simulink library "neural"  (Simulink 5.0)
undefined symbols (not defined in the file or in its folder): sfunxy2
libraries: simulink3 x7
settings Model: Creator=mani  LastModifiedBy=munlock -all d:\work\myr12\toolbox\fuzzy\fuzzy\mfedit.m

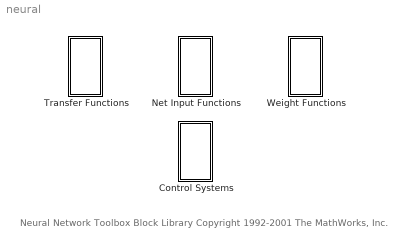
== system neural ==
  note: Neural Network Toolbox Block Library
      | Copyright 1992-2001 The MathWorks, Inc.
  Control Systems : Subsystem
      settings: RTWFcnNameOpts=Auto  RTWFileNameOpts=Auto
  Net Input Functions : Subsystem
      settings: RTWFcnNameOpts=Auto  RTWFileNameOpts=Auto
  Transfer Functions : Subsystem
      settings: RTWFcnNameOpts=Auto  RTWFileNameOpts=Auto
  Weight Functions : Subsystem
      settings: RTWFcnNameOpts=Auto  RTWFileNameOpts=Auto

== system neural/Control Systems ==
  Model Reference Controller : Subsystem  mask(NN Model Reference Control){Nrc=, Nic=, Njc=, IW_y=, IW_u=, IW_r=, B1_c=, B2_c=, LW_c=, retraining_c=, max_i_int=, min_i_int=, max_r_int=, min_r_int=, Ts=, S1=, Ni=, Nj=, sim_file=, trainfun=trainlm, Use_validation=, Use_Testing=, Use_Inc_training=, Use_previous_weights=, max_i=, min_i=, max_r=, min_r=, sam_training=, sam_training_c=, epochs=, epochs_c=, minp=, maxp=, mint=, maxt=, Normalize=, IW=, LW1_2=, LW2_1=, B1=, B2=, S1c=, Limit_output=, min_output=, max_output=, Ref_file=}
      mask prompts: Ts "Sample time"; trainfun "Training function Identification"; Limit_output "Limit output"
      mask help: Neural network model reference controller. You first train a neural network model of the plant to be controlled. Then train the controller so that the plant output will follow the output of a reference model. Double-click the Model Reference Control block to begin the plant and controller training.
      mask init:
      | xl = [0   .53     .53     .92   .92   .53   .53  NaN ];
      | yl = [.95 .95 1.05 1.05 .3   .3   .95 NaN  ];
      | x2 = [0 .53    NaN .92 1.2  ];
      | y2 = [.39 .39   NaN .65 .65  ];
      | t=(0:24)/24*2*pi;
      | xs = .07*cos(t)+.9;
      | ys = .07*sin(t)+.75;
      | 
      | x1t=.03; y1t=.31;
      | x2t=.03; y2t=.8;
      | x3t=.77; y3t=.53;
      | x4t=.77; y4t=.44;
      | x5t=.45; y5t=.66;
      | x6t=.45; y6t=.55;
      | x7t=.45; y7t=.44;
      settings: OpenFcn=nncontrolutil('nnmodref','',gcbh,gcb,'');  RTWFcnNameOpts=Auto  RTWFileNameOpts=Auto
      mask Help: eval('nnetbhelp([],''contro10.html'')');
      mask StyleString: edit,edit,edit,edit,edit,edit,edit,edit,edit,edit,edit,edit,edit,edit,edit,edit,edit,edit,edit,popup(trainbfg|trainbr |traincgb|traincgf|traincgp|traingd|traingdm|traingda|traingdx|trainlm |trainoss|trainrp |trainscg),edit,edit,edit,edit,edit,edit,edit,edit,edit,edit,edit,edit,edit,edit,edit,edit,edit,edit,edit,edit,edit,edit,edit,edit,edit,edit,edit
      mask Display:
      | plot([[xl NaN x2]*.9-.075 ], [[yl  NaN y2]*.9-.1 ]);
      | text(x1t,y1t,'Plant Output');
      | text(x2t,y2t,'Reference');
      | text(x3t,y3t,'Control');
      | text(x4t,y4t,'Signal');
      | text(x5t,y5t,'Neural');
      | text(x6t,y6t,'Network');
      | text(x7t,y7t,'Controller');
  NARMA-L2 Controller : Subsystem  mask(NARMA-L2 Controller){Normalize=, IW1_1=, IW3_2=, IW5_3=, LW2_1=, LW4_3=, LW5_4=, LW6_5=, LW6_2=, B1=, B2=, B3=, B4=, Limit_output=, min_output=, max_output=, Use_Previous_Weights=, Ts=, S1=, Ni=, Nj=, sim_file=, trainfun=trainlm, Use_validation=, Use_Testing=, max_i=, min_i=, max_i_int=, min_i_int=, sam_training=, epochs=, minp=, maxp=, mint=, maxt=}
      mask prompts: Ts "Sample time"; trainfun "Training function"
      mask help: NARMA-L2 Controller. You first train a neural network model of the plant to be controlled. The controller is a rearrangement of the trained plant model. Double-click the NARMA-L2 Controller block to begin the plant training.
      mask init:
      | xl = [0    .4   NaN  .33  .55   .55  .33  .33  NaN .80  .92 .92];
      | yl = [.95 .95 NaN  .75  .75   .55  .55  .75  NaN  .95 .95 .65];
      | x2 = [0    .43 NaN .45 .45    NaN .92 1.2 NaN .63 .85 .85 .63 .63 ];
      | y2 = [.39 .39 NaN  .41 .55   NaN .65 .65 NaN .75 .75  .55  .55  .75];
      | x3 = [.45 .45 NaN .42 .45 .48  NaN .33 .4 .33];
      | y3 = [.75 .90 NaN .83 .90 .83  NaN  .98 .95 .92];
      | x4 = [.75 .75 NaN .72 .75 .78  NaN  .5 .7 NaN .63 .7 .63];
      | y4 = [.75 .90 NaN .83 .90 .83  NaN .95 .95 NaN .98 .95 .92];
      | x5 = [.43 .43 .77 .77 .43 NaN .36 .43 .36 NaN .75 .75];
      | y5 = [.37 .41 .41 .37 .37 NaN .42 .39 .36 NaN .41 .55];
      | x6 = [.92 .92 .77 NaN .84 .77 .84];
      | y6 = [.65 .39 .39 NaN .42 .39 .36];
      | x1t=.03; y1t=.31;
      | x2t=.03; y2t=.85;
      | x8t=.03;y8t=.21;
      | x3t=.77; y3t=.53;
      | x4t=.77; y4t=.44;
      | x5t=.34; y5t=.49;
      | x6t=.58; y6t=.49;
      | 
      | 
      | t=(0:24)/24*2*pi;
      | xs = .05*cos(t);
      | ys = .05*sin(t);
      | xs1=xs+.45;
      | ys1=ys+.95;
      | xs2=xs+.75;
      | ys2=ys+.95;
      settings: OpenFcn=nncontrolutil('nnident','',gcbh,gcb,'narma_l2');  RTWFcnNameOpts=Auto  RTWFileNameOpts=Auto
      mask Help: eval('nnetbhelp([],''contro6a.html'')');
      mask StyleString: edit,edit,edit,edit,edit,edit,edit,edit,edit,edit,edit,edit,edit,edit,edit,edit,edit,edit,edit,edit,edit,edit,popup(trainbfg|trainbr |traincgb|traincgf|traincgp|traingd|traingdm|traingda|traingdx|trainlm |trainoss|trainrp |trainscg),edit,edit,edit,edit,edit,edit,edit,edit,edit,edit,edit,edit
      mask Display:
      | plot([[xl NaN x2]*.9-.075 ], [[yl  NaN y2]*.9-.1 ]);
      | plot([[x3 NaN xs1 NaN xs2]*.9-.075 ], [[y3 NaN ys1 NaN ys2]*.9-.1 ]);
      | plot([x4 NaN x5]*.9-.075,[y4 NaN y5]*.9-.1);
      | plot([x6 NaN ]*.9-.075,[y6 NaN ]*.9-.1);
      | text(x1t,y1t,'Plant');
      | text(x8t,y8t,'Output');
      | text(x2t,y2t,'Reference');
      | text(x3t,y3t,'Control');
      | text(x4t,y4t,'Signal');
      | text(x5t,y5t,'f');
      | text(x6t,y6t,'g');
  NN Predictive Controller : Subsystem  mask(NN Predictive Controller){epochs=, minp=, maxp=, mint=, maxt=, Normalize=, IW=, LW1_2=, LW2_1=, B1=, B2=, max_i_int=, min_i_int=, limit_output=, max_output=, min_output=, Use_Previous_Weights=, N2=, Nu=, Ts=, rho=, alpha=, csrchfun=csrchbac, maxiter=, S1=, Ni=, Nj=, sim_file=, trainfun=trainlm, Use_validation=, Use_Testing=, max_i=, min_i=, sam_training=}
      mask prompts: Ts "Sample time"; rho "rho (typically = 0.03)"; alpha "alpha (typically = 0.001)"; csrchfun "Minimization rutine"; trainfun "Training function"
      mask help: NN Predictive Controller. You first train a neural network model of the plant to be controlled. The controller uses the plant model to predict plant performance over a specified time horizon. An optimization algorithm determines the control signal that optimizes plant performance over this horizon. Double click the NN Predictive Controller block to train the plant model and set the controller parameters.
      mask init:
      | xl = [0   .53   .53     .85   .85  .53  .53  NaN .85  .92 .92];
      | yl = [.95 .95 1.05  1.05   .82  .82  .95  NaN  .95 .95 .65];
      | x2 = [0 .53    NaN .92 1.2 NaN .53 .85 .85 .53 .53 ];
      | y2 = [.39 .39   NaN .65 .65 NaN .59 .59 .29 .29  .59];
      | x3 = [.67 .67 NaN .64 .67 .70 NaN .53 .4   .4   .53 NaN .46 .53 .46];
      | y3 = [.59 .82 NaN .66 .59 .66 NaN .55 .55 .86 .86 NaN  .89 .86 .83];
      | 
      | x1t=.03; y1t=.31;
      | x2t=.03; y2t=.8;
      | x8t=.03;y8t=.21;
      | x3t=.77; y3t=.53;
      | x4t=.77; y4t=.44;
      | x5t=.45; y5t=.76;
      | x6t=.45; y6t=.35;
      | x7t=.45; y7t=.25;
      settings: OpenFcn=nncontrolutil('nnpredict','',gcbh,gcb);  RTWFcnNameOpts=Auto  RTWFileNameOpts=Auto
      mask Help: eval('nnetbhelp([],''control2.html'')');
      mask StyleString: edit,edit,edit,edit,edit,edit,edit,edit,edit,edit,edit,edit,edit,edit,edit,edit,edit,edit,edit,edit,edit,edit,popup(csrchgol|csrchbac|csrchhyb|csrchbre|csrchcha),edit,edit,edit,edit,edit,popup(trainbfg|trainbr |traincgb|traincgf|traincgp|traingd|traingdm|traingda|traingdx|trainlm |trainoss|trainrp |trainscg),edit,edit,edit,edit,edit
      mask Display:
      | plot([[xl NaN x2]*.9-.075 ], [[yl  NaN y2]*.9-.1 ]);
      | plot([[x3]*.9-.075 ], [[y3]*.9-.1 ]);
      | text(x1t,y1t,'Plant');
      | text(x8t,y8t,'Output');
      | text(x2t,y2t,'Reference');
      | text(x3t,y3t,'Control');
      | text(x4t,y4t,'Signal');
      | text(x5t,y5t,'Optim.');
      | text(x6t,y6t,'NN');
      | text(x7t,y7t,'Model');
  X(2Y)  Graph : Subsystem  LoadFcn=sfunxy2([],[],[],'LoadBlock')  StartFcn=sfunxy2([],[],[],'Start')  StopFcn=sfunxy2([],[],[],'Stop')  mask(X(2Y) scope.){xmin=0, xmax=5, ymin=21, ymax=22, st=-1}
      mask prompts: xmin "x-min:"; xmax "x-max:"; ymin "y-min:"; ymax "y-max:"; st "Sample time:"
      mask help: X(2Y) scope using MATLAB graph window. First input is used as time base. Enter plotting ranges.
      settings: CopyFcn=sfunxy2([],[],[],'CopyBlock')  DeleteFcn=sfunxy2([],[],[],'DeleteBlock')  NameChangeFcn=sfunxy2([],[],[],'NameChange')  RTWFcnNameOpts=Auto  RTWFileNameOpts=Auto
      mask Help: This block can be used to explore limit cycles. Look at the m-file sfunxy.m to see how it works.
      mask Display: plot([.05 .95 .95 .05 .05],[.45 .45 .95 .95 .45], 0.5+cos(0:0.1:2*pi)*0.3,0.7+sin(0:0.1:2*pi)*0.2)

== system neural/Net Input Functions ==
  netprod : Product  Inputs=2  Multiplication=Element-wise(.*)  SaturateOnIntegerOverflow=on
  netsum : Sum  Inputs=2  SaturateOnIntegerOverflow=on

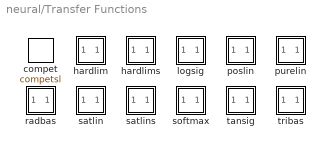
== system neural/Transfer Functions ==
  compet : MATLABFcn  MATLABFcn=competsl  OutputDimensions=-1  OutputSignalType=auto  Output1D=on
      mask Type: compet
      mask Description: Competitive transfer function
      mask Help: eval('nnetbhelp(''compet'')');
      mask Display: disp('C')
  hardlim : Subsystem
      settings: RTWFcnNameOpts=Auto  RTWFileNameOpts=Auto
      mask Type: Hardlim
      mask Description: Hard limit transfer function
      mask Help: eval('nnetbhelp(''hardlim'')');
      mask Display: plot([-1 1],[-1 -1],[-1 0 0 1],[-1 -1 1 1])
  hardlims : Subsystem
      settings: RTWFcnNameOpts=Auto  RTWFileNameOpts=Auto
      mask Description: Symmetric hard limit transfer function
      mask Help: eval('nnetbhelp(''hardlims'')');
      mask Display: plot([-1 1],[0 0],[-1 0 0 1],[-1 -1 1 1])
  logsig : Subsystem
      settings: RTWFcnNameOpts=Auto  RTWFileNameOpts=Auto
      mask Description: Log sigmoid transfer function
      mask Help: eval('nnetbhelp(''logsig'')');
      mask Display: plot([-1 1],[0 0],[-1 -.9 -.8 -.7 -.6 -.5 -.4 -.3 -.2 -.1 0 .1 .2 .3 .4 .5 .6 .7 .8 .9 1],1./(1+exp(-8*[-1 -.9 -.8 -.7 -.6 -.5 -.4 -.3 -.2 -.1 0 .1 .2 .3 .4 .5 .6 .7 .8 .9 1]))+.01)
  poslin : Subsystem  Orientation=left
      settings: RTWFcnNameOpts=Auto  RTWFileNameOpts=Auto
      mask Description: Positive linear transfer function
      mask Help: eval('nnetbhelp(''poslin'')');
      mask Display: plot([-1 1],[-1 -1],[-1 -.5 1],[-1 -1 1])
  purelin : Subsystem
      settings: RTWFcnNameOpts=Auto  RTWFileNameOpts=Auto
      mask Description: Linear transfer function
      mask Help: eval('nnetbhelp(''purelin'')');
      mask Display: plot([-1 1],[0 0],[-1 1],[-1 1])
  radbas : Subsystem
      settings: RTWFcnNameOpts=Auto  RTWFileNameOpts=Auto
      mask Description: Radial basis transfer function
      mask Help: eval('nnetbhelp(''radbas'')');
      mask Display: plot([-1 1],[0 0],[-1 -.9 -.8 -.7 -.6 -.5 -.4 -.3 -.2 -.1 0 .1 .2 .3 .4 .5 .6 .7 .8 .9 1],exp(-4*([-1 -.9 -.8 -.7 -.6 -.5 -.4 -.3 -.2 -.1 0 .1 .2 .3 .4 .5 .6 .7 .8 .9 1].^2)))
  satlin : Subsystem
      settings: RTWFcnNameOpts=Auto  RTWFileNameOpts=Auto
      mask Description: Saturating linear transfer function
      mask Help: eval('nnetbhelp(''satlin'')');
      mask Display: plot([-1 1],[-1 -1],[-1 -0.5 0.5 1],[-1 -1 1 1])
  satlins : Subsystem
      settings: RTWFcnNameOpts=Auto  RTWFileNameOpts=Auto
      mask Description: Symmetric saturating linear transfer function
      mask Help: eval('nnetbhelp(''satlins'')');
      mask Display: plot([-1 1],[0 0],[-1 -0.5 0.5 1],[-1 -1 1 1])
  softmax : Subsystem
      settings: RTWFcnNameOpts=Auto  RTWFileNameOpts=Auto
      mask Description: Soft max transfer function
      mask Help: eval('nnetbhelp(''softmax'')');
      mask Display: disp('S')
  tansig : Subsystem
      settings: RTWFcnNameOpts=Auto  RTWFileNameOpts=Auto
      mask Description: Hyperbolic tangent sigmoid transfer function
      mask Help: eval('nnetbhelp(''tansig'')');
      mask Display: plot([-1 1],[0 0],[-1 -.9 -.8 -.7 -.6 -.5 -.4 -.3 -.2 -.1 0 .1 .2 .3 .4 .5 .6 .7 .8 .9 1],2./(1+exp(-8*[-1 -.9 -.8 -.7 -.6 -.5 -.4 -.3 -.2 -.1 0 .1 .2 .3 .4 .5 .6 .7 .8 .9 1]))-1)
  tribas : Subsystem
      settings: RTWFcnNameOpts=Auto  RTWFileNameOpts=Auto
      mask Description: Triangular basis transfer function
      mask Help: eval('nnetbhelp(''tribas'')');
      mask Display: plot([-1 1],[0 0],[-1 -.6 0 .6 1],[0 0 1 0 0])

== system neural/Weight Functions ==
  dist : Subsystem
      settings: RTWFcnNameOpts=Auto  RTWFileNameOpts=Auto
      mask Description: Euclidean distance weight function
      mask Help: eval('nnetbhelp(''dist'')');
  dotprod : Subsystem
      settings: RTWFcnNameOpts=Auto  RTWFileNameOpts=Auto
      mask Description: Dot product weight function
      mask Help: eval('nnetbhelp(''dotprod'')');
  negdist : Subsystem
      settings: RTWFcnNameOpts=Auto  RTWFileNameOpts=Auto
      mask Description: The negative of the euclidean distance weight function
      mask Help: eval('nnetbhelp(''negdist'')');
  normprod : Subsystem
      settings: RTWFcnNameOpts=Auto  RTWFileNameOpts=Auto
      mask Description: Normalized dot product weight function
      mask Help: eval('nnetbhelp(''normprod'')');

== system neural/Control Systems/Model Reference Controller ==
  Reference : Inport  Port=1  LatchInput=off
  Plant Output : Inport  Orientation=up  Port=2  LatchInput=off
  NN Controller : Subsystem
      settings: RTWFcnNameOpts=Auto  RTWFileNameOpts=Auto
  NN Plant : Subsystem
      settings: RTWFcnNameOpts=Auto  RTWFileNameOpts=Auto
  Terminator : Terminator
  Terminator1 : Terminator
  Control Signal : Outport  Orientation=down  Port=1
  wires:
  NN Plant/2(yhat1) -> Terminator1/1
  NN Plant/1(yhat) -> Terminator/1
  Reference/1 -> NN Controller/1(r)
  NN Controller/1(uhat) -> NN Controller/2(u), Control Signal/1, NN Plant/1(u)
  Plant Output/1 -> NN Controller/3(y), NN Plant/2(y)

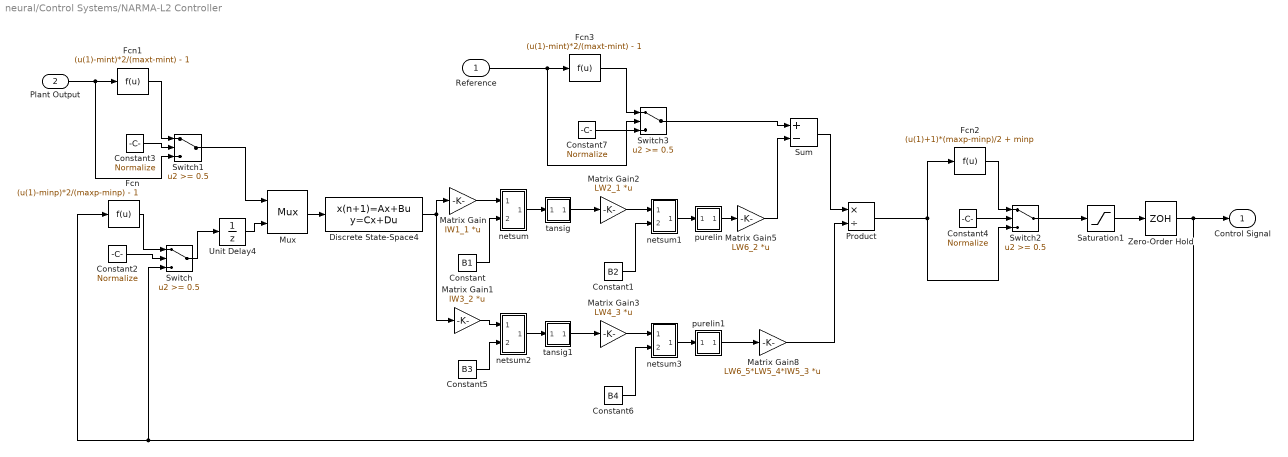
== system neural/Control Systems/NARMA-L2 Controller ==
  Reference : Inport  Port=1  LatchInput=off
  Plant Output : Inport  Port=2  LatchInput=off
  Constant : Constant  Value=B1
  Constant1 : Constant  Value=B2
  Constant{2..4,7} (4 alike) : Constant  Value=Normalize
  Constant5 : Constant  Value=B3
  Constant6 : Constant  Value=B4
  Discrete State-Space4 : DiscreteStateSpace  A=blkdiag([zeros(1,Nj-1);eye(Nj-2,Nj-2) zeros(Nj-2,1)],[zeros(1,Ni-1);eye(Ni-2,Ni-2) zeros(Ni-2,1)])  B=blkdiag(eye(Nj-1,1),eye(Ni-1,1))  C=blkdiag([zeros(1,Nj-1);eye(Nj-1,Nj-1)],[zeros(eye(double(Ni>1)),Ni-1);eye(Ni-2,Ni-1)])  D=blkdiag([1;zeros(Nj-1,1)],[eye(double(Ni>1));zeros(Ni-2,1)])  X0=0  SampleTime=Ts  Realization=auto
      settings: RTWStateStorageClass=Auto
  Fcn : Fcn  Expr=(u(1)-minp)*2/(maxp-minp) - 1
  Fcn1 : Fcn  Expr=(u(1)-mint)*2/(maxt-mint) - 1
  Fcn2 : Fcn  Expr=(u(1)+1)*(maxp-minp)/2 + minp
  Fcn3 : Fcn  Expr=(u(1)-mint)*2/(maxt-mint) - 1
  Matrix Gain : Gain  Gain=IW1_1  Multiplication=Matrix(K*u)  SaturateOnIntegerOverflow=on
  Matrix Gain1 : Gain  Gain=IW3_2  Multiplication=Matrix(K*u)  SaturateOnIntegerOverflow=on
  Matrix Gain2 : Gain  Gain=LW2_1  Multiplication=Matrix(K*u)  SaturateOnIntegerOverflow=on
  Matrix Gain3 : Gain  Gain=LW4_3  Multiplication=Matrix(K*u)  SaturateOnIntegerOverflow=on
  Matrix Gain5 : Gain  Gain=LW6_2  Multiplication=Matrix(K*u)  SaturateOnIntegerOverflow=on
  Matrix Gain8 : Gain  Gain=LW6_5*LW5_4*IW5_3  Multiplication=Matrix(K*u)  SaturateOnIntegerOverflow=on
  Mux : Mux  Inputs=2
      settings: DisplayOption=signals
  Product : Product  Inputs=*/  Multiplication=Element-wise(.*)  SaturateOnIntegerOverflow=on
  Saturation1 : Saturate  UpperLimit=max_i  LowerLimit=min_i  LinearizeAsGain=on  ZeroCross=off
  Sum : Sum  Inputs=+-  SaturateOnIntegerOverflow=on
  Switch{,1..3} (4 alike) : Switch  Threshold=0.5  ZeroCross=off
  Unit Delay4 : UnitDelay  X0=0  SampleTime=Ts
      settings: RTWStateStorageClass=Auto
  Zero-Order Hold : ZeroOrderHold  SampleTime=Ts
  netsum : Subsystem
      settings: RTWFcnNameOpts=Auto  RTWFileNameOpts=Auto
      mask Display: disp('+')
  netsum1 : Subsystem
      settings: RTWFcnNameOpts=Auto  RTWFileNameOpts=Auto
      mask Display: disp('+')
  netsum2 : Subsystem
      settings: RTWFcnNameOpts=Auto  RTWFileNameOpts=Auto
      mask Display: disp('+')
  netsum3 : Subsystem
      settings: RTWFcnNameOpts=Auto  RTWFileNameOpts=Auto
      mask Display: disp('+')
  purelin : Subsystem
      settings: RTWFcnNameOpts=Auto  RTWFileNameOpts=Auto
      mask Display: plot([-1 1],[0 0],[-1 1],[-1 1])
  purelin1 : Subsystem
      settings: RTWFcnNameOpts=Auto  RTWFileNameOpts=Auto
      mask Display: plot([-1 1],[0 0],[-1 1],[-1 1])
  tansig : Subsystem
      settings: RTWFcnNameOpts=Auto  RTWFileNameOpts=Auto
      mask Display: plot([-1 1],[0 0],[-1 -.9 -.8 -.7 -.6 -.5 -.4 -.3 -.2 -.1 0 .1 .2 .3 .4 .5 .6 .7 .8 .9 1],2./(1+exp(-8*[-1 -.9 -.8 -.7 -.6 -.5 -.4 -.3 -.2 -.1 0 .1 .2 .3 .4 .5 .6 .7 .8 .9 1]))-1)
  tansig1 : Subsystem
      settings: RTWFcnNameOpts=Auto  RTWFileNameOpts=Auto
      mask Display: plot([-1 1],[0 0],[-1 -.9 -.8 -.7 -.6 -.5 -.4 -.3 -.2 -.1 0 .1 .2 .3 .4 .5 .6 .7 .8 .9 1],2./(1+exp(-8*[-1 -.9 -.8 -.7 -.6 -.5 -.4 -.3 -.2 -.1 0 .1 .2 .3 .4 .5 .6 .7 .8 .9 1]))-1)
  Control Signal : Outport  Port=1
  wires:
  Saturation1/1 -> Zero-Order Hold/1
  Switch/1 -> Unit Delay4/1
  Unit Delay4/1 -> Mux/2
  Constant2/1 -> Switch/2
  Fcn/1 -> Switch/1
  Zero-Order Hold/1 -> Switch/3, Fcn/1, Control Signal/1
  Discrete State-Space4/1 -> Matrix Gain1/1, Matrix Gain/1
  Mux/1 -> Discrete State-Space4/1
  Switch1/1 -> Mux/1
  Switch3/1 -> Sum/1
  Reference/1 -> Switch3/3, Fcn3/1
  Fcn3/1 -> Switch3/1
  Constant7/1 -> Switch3/2
  Matrix Gain8/1 -> Product/2
  purelin1/1(a) -> Matrix Gain8/1
  Sum/1 -> Product/1
  Matrix Gain5/1 -> Sum/2
  purelin/1(a) -> Matrix Gain5/1
  Matrix Gain1/1 -> netsum2/1(In1)
  tansig1/1(a) -> Matrix Gain3/1
  Constant5/1 -> netsum2/2(In2)
  netsum2/1(Out1) -> tansig1/1(n)
  Matrix Gain3/1 -> netsum3/1(In1)
  Constant6/1 -> netsum3/2(In2)
  netsum3/1(Out1) -> purelin1/1(n)
  Matrix Gain/1 -> netsum/1(In1)
  tansig/1(a) -> Matrix Gain2/1
  Constant/1 -> netsum/2(In2)
  netsum/1(Out1) -> tansig/1(n)
  Matrix Gain2/1 -> netsum1/1(In1)
  Constant1/1 -> netsum1/2(In2)
  netsum1/1(Out1) -> purelin/1(n)
  Plant Output/1 -> Switch1/3, Fcn1/1
  Fcn1/1 -> Switch1/1
  Constant3/1 -> Switch1/2
  Product/1 -> Fcn2/1, Switch2/3
  Constant4/1 -> Switch2/2
  Switch2/1 -> Saturation1/1
  Fcn2/1 -> Switch2/1

== system neural/Control Systems/NN Predictive Controller ==
  Reference : Inport  Orientation=down  Port=1  LatchInput=off
  Plant output : Inport  Orientation=up  Port=2  LatchInput=off
  Mux : Mux  Orientation=down  Inputs=4
      settings: DisplayOption=signals
  NN model : Subsystem
      settings: RTWFcnNameOpts=Auto  RTWFileNameOpts=Auto
  S-Function : S-Function  Orientation=down  FunctionName=predopt  Parameters=N2,Ts,Nu,maxiter,csrchfun,rho,alpha,S1,IW,LW1_2,LW2_1,B1,B2,Ni,Nj,min_i,max_i,minp,maxp,mint,maxt,Normalize  PortCounts=[]  SFunctionModules=''
  Control Signal : Outport  Orientation=down  Port=1
  wires:
  Plant output/1 -> Mux/2, NN model/2(y)
  Reference/1 -> Mux/1
  NN model/1(yhat) -> Mux/3
  NN model/2(yhat1) -> Mux/4
  S-Function/1 -> Control Signal/1, NN model/1(u)
  Mux/1 -> S-Function/1

== system neural/Control Systems/X(2Y)  Graph ==
  x : Inport  Port=1  LatchInput=off
  y1 : Inport  Port=2  LatchInput=off
  y2 : Inport  Port=3  LatchInput=off
  Mux : Mux  Inputs=3
      settings: DisplayOption=none
  sfunxy : S-Function  FunctionName=sfunxy2  Parameters=[xmin xmax ymin ymax], st  PortCounts=[]  SFunctionModules=''
  wires:
  y2/1 -> Mux/3
  y1/1 -> Mux/2
  x/1 -> Mux/1
  Mux/1 -> sfunxy/1

== system neural/Transfer Functions/hardlim ==
  n : Inport  Port=1  LatchInput=off
  Constant : Constant  Value=0.5
  Gain : Gain  Gain=0.5  Multiplication=Element-wise(K.*u)  SaturateOnIntegerOverflow=on
  Sign : Signum  ZeroCross=off
  Sum : Sum  Inputs=++  SaturateOnIntegerOverflow=on
  a : Outport  Port=1  InitialOutput=0
  wires:
  Sum/1 -> a/1
  n/1 -> Sign/1
  Constant/1 -> Sum/2
  Gain/1 -> Sum/1
  Sign/1 -> Gain/1

== system neural/Transfer Functions/hardlims ==
  n : Inport  Port=1  LatchInput=off
  Sign : Signum  ZeroCross=off
  a : Outport  Port=1  InitialOutput=0
  wires:
  n/1 -> Sign/1
  Sign/1 -> a/1

== system neural/Transfer Functions/logsig ==
  n : Inport  Port=1  LatchInput=off
  Exp : ElementaryMath  Operator=exp
  Gain : Gain  Gain=-1  Multiplication=Element-wise(K.*u)  SaturateOnIntegerOverflow=on
  Reciprocal : ElementaryMath  Operator=reciprocal
  Sum : Sum  Inputs=++  SaturateOnIntegerOverflow=on
  one : Constant  Value=1
  a : Outport  Port=1  InitialOutput=0
  wires:
  Reciprocal/1 -> a/1
  Sum/1 -> Reciprocal/1
  one/1 -> Sum/2
  Exp/1 -> Sum/1
  Gain/1 -> Exp/1
  n/1 -> Gain/1

== system neural/Transfer Functions/poslin ==
  n : Inport  Port=1  LatchInput=off
  Saturation : Saturate  UpperLimit=inf  LowerLimit=0  LinearizeAsGain=on  ZeroCross=off
  a : Outport  Port=1  InitialOutput=0
  wires:
  n/1 -> Saturation/1
  Saturation/1 -> a/1

== system neural/Transfer Functions/purelin ==
  n : Inport  Port=1  LatchInput=off
  a : Outport  Port=1  InitialOutput=0
  wires:
  n/1 -> a/1

== system neural/Transfer Functions/radbas ==
  n : Inport  Port=1  LatchInput=off
  Exp : ElementaryMath  Operator=exp
  Gain : Gain  Gain=-1  Multiplication=Element-wise(K.*u)  SaturateOnIntegerOverflow=on
  Product : Product  Inputs=2  Multiplication=Element-wise(.*)  SaturateOnIntegerOverflow=on
  a : Outport  Port=1  InitialOutput=0
  wires:
  Exp/1 -> a/1
  Gain/1 -> Exp/1
  Product/1 -> Gain/1
  n/1 -> Product/2, Product/1

== system neural/Transfer Functions/satlin ==
  n : Inport  Port=1  LatchInput=off
  Saturation : Saturate  UpperLimit=1  LowerLimit=0  LinearizeAsGain=on  ZeroCross=off
  a : Outport  Port=1  InitialOutput=0
  wires:
  n/1 -> Saturation/1
  Saturation/1 -> a/1

== system neural/Transfer Functions/satlins ==
  n : Inport  Port=1  LatchInput=off
  Saturation : Saturate  UpperLimit=1  LowerLimit=-1  LinearizeAsGain=on  ZeroCross=off
  a : Outport  Port=1  InitialOutput=0
  wires:
  n/1 -> Saturation/1
  Saturation/1 -> a/1

== system neural/Transfer Functions/softmax ==
  n : Inport  Port=1  LatchInput=off
  Exp : ElementaryMath  Operator=exp
  Product : Product  Inputs=2  Multiplication=Element-wise(.*)  SaturateOnIntegerOverflow=on
  Reciprocal : ElementaryMath  Operator=reciprocal
  Sum : Sum  Inputs=+  SaturateOnIntegerOverflow=on
  a : Outport  Port=1  InitialOutput=0
  wires:
  Product/1 -> a/1
  Exp/1 -> Product/2, Sum/1
  Reciprocal/1 -> Product/1
  Sum/1 -> Reciprocal/1
  n/1 -> Exp/1

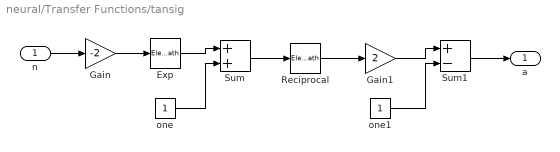
== system neural/Transfer Functions/tansig ==
  n : Inport  Port=1  LatchInput=off
  Exp : ElementaryMath  Operator=exp
  Gain : Gain  Gain=-2  Multiplication=Element-wise(K.*u)  SaturateOnIntegerOverflow=on
  Gain1 : Gain  Gain=2  Multiplication=Element-wise(K.*u)  SaturateOnIntegerOverflow=on
  Reciprocal : ElementaryMath  Operator=reciprocal
  Sum : Sum  Inputs=++  SaturateOnIntegerOverflow=on
  Sum1 : Sum  Inputs=+-  SaturateOnIntegerOverflow=on
  one : Constant  Value=1
  one1 : Constant  Value=1
  a : Outport  Port=1  InitialOutput=0
  wires:
  Sum1/1 -> a/1
  one1/1 -> Sum1/2
  Gain1/1 -> Sum1/1
  Reciprocal/1 -> Gain1/1
  Sum/1 -> Reciprocal/1
  one/1 -> Sum/2
  Exp/1 -> Sum/1
  Gain/1 -> Exp/1
  n/1 -> Gain/1

== system neural/Transfer Functions/tribas ==
  In1 : Inport  Port=1  LatchInput=off
  Abs : Abs  SaturateOnIntegerOverflow=on  ZeroCross=off
  MinMax : MinMax  Function=max  Inputs=2  ZeroCross=off
  Sum : Sum  Inputs=+-  SaturateOnIntegerOverflow=on
  one : Constant  Value=1
  zero : Constant  Value=0
  Out1 : Outport  Port=1  InitialOutput=0
  wires:
  one/1 -> Sum/1
  In1/1 -> Abs/1
  Abs/1 -> Sum/2
  Sum/1 -> MinMax/1
  zero/1 -> MinMax/2
  MinMax/1 -> Out1/1

== system neural/Weight Functions/dist ==
  w : Inport  Port=1  LatchInput=off
  p : Inport  Port=2  LatchInput=off
  Diff : Sum  Inputs=+-  SaturateOnIntegerOverflow=on
  Product : Product  Inputs=2  Multiplication=Element-wise(.*)  SaturateOnIntegerOverflow=on
  Sqrt : ElementaryMath  Operator=sqrt
  Sum : Sum  Inputs=1  SaturateOnIntegerOverflow=on
  z : Outport  Port=1  InitialOutput=0
  wires:
  Sqrt/1 -> z/1
  Sum/1 -> Sqrt/1
  Product/1 -> Sum/1
  Diff/1 -> Product/2, Product/1
  p/1 -> Diff/2
  w/1 -> Diff/1

== system neural/Weight Functions/dotprod ==
  w : Inport  Port=1  LatchInput=off
  p : Inport  Port=2  LatchInput=off
  Dot Product : Subsystem  mask(Dot Product){}
      mask help:
      | Inner (dot) product.
      | y=sum(u1.*u2)
      mask init:
      | t=(0:.1:2*pi)';
      | x=cos(t);
      | y=sin(t);
      settings: RTWFcnNameOpts=Auto  RTWFileNameOpts=Auto
      mask Help: Computes the inner (dot) product of the inputs: sum(u1.*u2).  The inputs are vectors of the same length. Output is a scalar.
      mask Display: plot(0,0,1,1,x*[0.025 0.07]+0.5,y*[0.025 0.07]+0.5)
  z : Outport  Port=1  InitialOutput=0
  wires:
  Dot Product/1(out_1) -> z/1
  p/1 -> Dot Product/2(in_2)
  w/1 -> Dot Product/1(in_1)

== system neural/Weight Functions/negdist ==
  w : Inport  Port=1  LatchInput=off
  p : Inport  Port=2  LatchInput=off
  Diff : Sum  Inputs=+-  SaturateOnIntegerOverflow=on
  Gain : Gain  Gain=-1  Multiplication=Element-wise(K.*u)  SaturateOnIntegerOverflow=on
  Product : Product  Inputs=2  Multiplication=Element-wise(.*)  SaturateOnIntegerOverflow=on
  Sqrt : ElementaryMath  Operator=sqrt
  Sum : Sum  Inputs=1  SaturateOnIntegerOverflow=on
  z : Outport  Port=1  InitialOutput=0
  wires:
  Gain/1 -> z/1
  Sqrt/1 -> Gain/1
  Sum/1 -> Sqrt/1
  Product/1 -> Sum/1
  Diff/1 -> Product/2, Product/1
  p/1 -> Diff/2
  w/1 -> Diff/1

== system neural/Weight Functions/normprod ==
  w : Inport  Port=1  LatchInput=off
  p : Inport  Port=2  LatchInput=off
  Dot Product : Subsystem  mask(Dot Product){}
      mask help:
      | Inner (dot) product.
      | y=sum(u1.*u2)
      mask init:
      | t=(0:.1:2*pi)';
      | x=cos(t);
      | y=sin(t);
      settings: RTWFcnNameOpts=Auto  RTWFileNameOpts=Auto
      mask Help: Computes the inner (dot) product of the inputs: sum(u1.*u2).  The inputs are vectors of the same length. Output is a scalar.
      mask Display: plot(0,0,1,1,x*[0.025 0.07]+0.5,y*[0.025 0.07]+0.5)
  Product : Product  Inputs=2  Multiplication=Element-wise(.*)  SaturateOnIntegerOverflow=on
  Reciprocal : ElementaryMath  Operator=reciprocal
  Sum : Sum  Inputs=1  SaturateOnIntegerOverflow=on
  z : Outport  Port=1  InitialOutput=0
  wires:
  Product/1 -> z/1
  Reciprocal/1 -> Product/2
  Dot Product/1(out_1) -> Product/1
  Sum/1 -> Reciprocal/1
  p/1 -> Dot Product/2(in_2), Sum/1
  w/1 -> Dot Product/1(in_1)

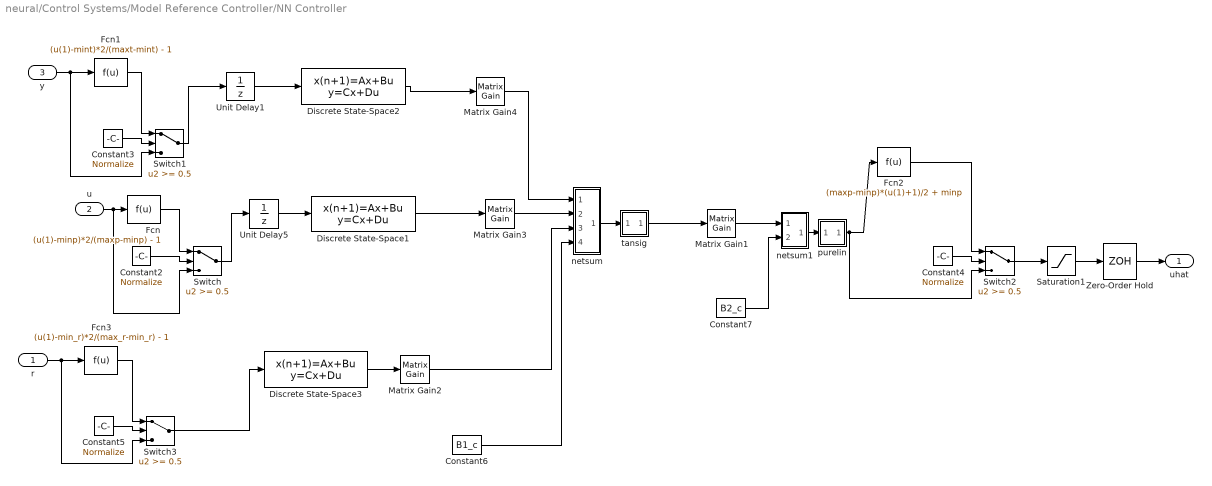
== system neural/Control Systems/Model Reference Controller/NN Controller ==
  r : Inport  Port=1  LatchInput=off
  u : Inport  Port=2  LatchInput=off
  y : Inport  Port=3  LatchInput=off
  Constant{2..5} (4 alike) : Constant  Value=Normalize
  Constant6 : Constant  Value=B1_c
  Constant7 : Constant  Value=B2_c
  Discrete State-Space1 : DiscreteStateSpace  A=[zeros(1,max([Nic-1 1]));eye(Nic-2,Nic-1)]  B=eye(max([Nic-1 1]),1)  C=[zeros(1,max([Nic-1 1]));eye(Nic-1,Nic-1)]  D=eye(Nic,1)  X0=0  SampleTime=Ts  Realization=auto
      settings: RTWStateStorageClass=Auto
  Discrete State-Space2 : DiscreteStateSpace  A=[zeros(1,max([Njc-1 1]));eye(Njc-2,Njc-1)]  B=eye(max([Njc-1 1]),1)  C=[zeros(1,max([Njc-1 1]));eye(Njc-1,Njc-1)]  D=eye(Njc,1)  X0=0  SampleTime=Ts  Realization=auto
      settings: RTWStateStorageClass=Auto
  Discrete State-Space3 : DiscreteStateSpace  A=[zeros(1,max([Nrc-1 1]));eye(Nrc-2,Nrc-1)]  B=eye(max([Nrc-1 1]),1)  C=[zeros(1,max([Nrc-1 1]));eye(Nrc-1,Nrc-1)]  D=eye(Nrc,1)  X0=0  SampleTime=Ts  Realization=auto
      settings: RTWStateStorageClass=Auto
  Fcn : Fcn  Expr=(u(1)-minp)*2/(maxp-minp) - 1
  Fcn1 : Fcn  Expr=(u(1)-mint)*2/(maxt-mint) - 1
  Fcn2 : Fcn  Expr=(maxp-minp)*(u(1)+1)/2 + minp
  Fcn3 : Fcn  Expr=(u(1)-min_r)*2/(max_r-min_r) - 1
  Matrix Gain1 : simulink3/Math/Matrix Gain  K=LW_c
  Matrix Gain2 : simulink3/Math/Matrix Gain  K=IW_r
  Matrix Gain3 : simulink3/Math/Matrix Gain  K=IW_u
  Matrix Gain4 : simulink3/Math/Matrix Gain  K=IW_y
  Saturation1 : Saturate  UpperLimit=max_i  LowerLimit=min_i  LinearizeAsGain=on  ZeroCross=off
  Switch{,1..3} (4 alike) : Switch  Threshold=0.5  ZeroCross=off
  Unit Delay1 : UnitDelay  X0=0  SampleTime=Ts
      settings: RTWStateStorageClass=Auto
  Unit Delay5 : UnitDelay  X0=0  SampleTime=Ts
      settings: RTWStateStorageClass=Auto
  Zero-Order Hold : ZeroOrderHold  SampleTime=Ts
  netsum : Subsystem
      settings: RTWFcnNameOpts=Auto  RTWFileNameOpts=Auto
      mask Display: disp('+')
  netsum1 : Subsystem
      settings: RTWFcnNameOpts=Auto  RTWFileNameOpts=Auto
      mask Display: disp('+')
  purelin : Subsystem
      settings: RTWFcnNameOpts=Auto  RTWFileNameOpts=Auto
      mask Display: plot([-1 1],[0 0],[-1 1],[-1 1])
  tansig : Subsystem
      settings: RTWFcnNameOpts=Auto  RTWFileNameOpts=Auto
      mask Display: plot([-1 1],[0 0],[-1 -.9 -.8 -.7 -.6 -.5 -.4 -.3 -.2 -.1 0 .1 .2 .3 .4 .5 .6 .7 .8 .9 1],2./(1+exp(-8*[-1 -.9 -.8 -.7 -.6 -.5 -.4 -.3 -.2 -.1 0 .1 .2 .3 .4 .5 .6 .7 .8 .9 1]))-1)
  uhat : Outport  Port=1
  wires:
  Fcn2/1 -> Switch2/1
  Fcn/1 -> Switch/1
  Discrete State-Space1/1 -> Matrix Gain3/1
  tansig/1(a) -> Matrix Gain1/1
  Discrete State-Space2/1 -> Matrix Gain4/1
  Switch3/1 -> Discrete State-Space3/1
  Unit Delay1/1 -> Discrete State-Space2/1
  Unit Delay5/1 -> Discrete State-Space1/1
  Saturation1/1 -> Zero-Order Hold/1
  Zero-Order Hold/1 -> uhat/1
  Discrete State-Space3/1 -> Matrix Gain2/1
  Constant7/1 -> netsum1/2(In2)
  Switch2/1 -> Saturation1/1
  purelin/1(a) -> Fcn2/1, Switch2/3
  Constant4/1 -> Switch2/2
  Matrix Gain1/1 -> netsum1/1(In1)
  netsum1/1(Out1) -> purelin/1(n)
  Matrix Gain2/1 -> netsum/3(In3)
  netsum/1(Out1) -> tansig/1(n)
  r/1 -> Switch3/3, Fcn3/1
  Fcn3/1 -> Switch3/1
  Constant5/1 -> Switch3/2
  y/1 -> Switch1/3, Fcn1/1
  Fcn1/1 -> Switch1/1
  Switch1/1 -> Unit Delay1/1
  Constant3/1 -> Switch1/2
  Constant2/1 -> Switch/2
  u/1 -> Fcn/1, Switch/3
  Switch/1 -> Unit Delay5/1
  Constant6/1 -> netsum/4(In4)
  Matrix Gain3/1 -> netsum/2(In2)
  Matrix Gain4/1 -> netsum/1(In1)

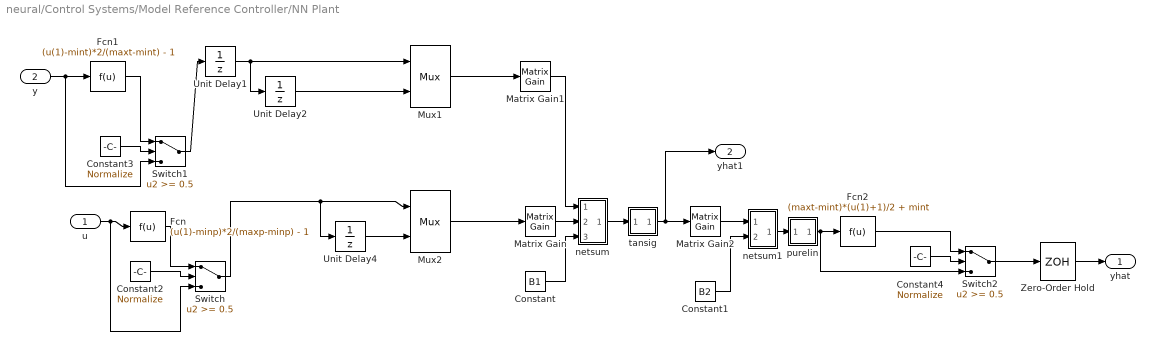
== system neural/Control Systems/Model Reference Controller/NN Plant ==
  u : Inport  Port=1  LatchInput=off
  y : Inport  Port=2  LatchInput=off
  Constant : Constant  Value=B1
  Constant1 : Constant  Value=B2
  Constant2 : Constant  Value=Normalize
  Constant3 : Constant  Value=Normalize
  Constant4 : Constant  Value=Normalize
  Fcn : Fcn  Expr=(u(1)-minp)*2/(maxp-minp) - 1
  Fcn1 : Fcn  Expr=(u(1)-mint)*2/(maxt-mint) - 1
  Fcn2 : Fcn  Expr=(maxt-mint)*(u(1)+1)/2 + mint
  Matrix Gain : simulink3/Math/Matrix Gain  K=IW
  Matrix Gain1 : simulink3/Math/Matrix Gain  K=LW1_2
  Matrix Gain2 : simulink3/Math/Matrix Gain  K=LW2_1
  Mux1 : Mux  Inputs=2
      settings: DisplayOption=signals
  Mux2 : Mux  Inputs=2
      settings: DisplayOption=signals
  Switch : Switch  Threshold=0.5  ZeroCross=off
  Switch1 : Switch  Threshold=0.5  ZeroCross=off
  Switch2 : Switch  Threshold=0.5  ZeroCross=off
  Unit Delay1 : UnitDelay  X0=0  SampleTime=Ts
      settings: RTWStateStorageClass=Auto
  Unit Delay2 : UnitDelay  X0=0  SampleTime=Ts
      settings: RTWStateStorageClass=Auto
  Unit Delay4 : UnitDelay  X0=0  SampleTime=Ts
      settings: RTWStateStorageClass=Auto
  Zero-Order Hold : ZeroOrderHold  SampleTime=Ts
  netsum : Subsystem
      settings: RTWFcnNameOpts=Auto  RTWFileNameOpts=Auto
      mask Display: disp('+')
  netsum1 : Subsystem
      settings: RTWFcnNameOpts=Auto  RTWFileNameOpts=Auto
      mask Display: disp('+')
  purelin : Subsystem
      settings: RTWFcnNameOpts=Auto  RTWFileNameOpts=Auto
      mask Display: plot([-1 1],[0 0],[-1 1],[-1 1])
  tansig : Subsystem
      settings: RTWFcnNameOpts=Auto  RTWFileNameOpts=Auto
      mask Display: plot([-1 1],[0 0],[-1 -.9 -.8 -.7 -.6 -.5 -.4 -.3 -.2 -.1 0 .1 .2 .3 .4 .5 .6 .7 .8 .9 1],2./(1+exp(-8*[-1 -.9 -.8 -.7 -.6 -.5 -.4 -.3 -.2 -.1 0 .1 .2 .3 .4 .5 .6 .7 .8 .9 1]))-1)
  yhat : Outport  Port=1
  yhat1 : Outport  Port=2
  wires:
  Switch2/1 -> Zero-Order Hold/1
  Zero-Order Hold/1 -> yhat/1
  Switch/1 -> Unit Delay4/1, Mux2/1
  Unit Delay4/1 -> Mux2/2
  Unit Delay2/1 -> Mux1/2
  Unit Delay1/1 -> Unit Delay2/1, Mux1/1
  y/1 -> Switch1/3, Fcn1/1
  Fcn1/1 -> Switch1/1
  Switch1/1 -> Unit Delay1/1
  Constant3/1 -> Switch1/2
  Mux1/1 -> Matrix Gain1/1
  Constant2/1 -> Switch/2
  u/1 -> Switch/3, Fcn/1
  Fcn/1 -> Switch/1
  Mux2/1 -> Matrix Gain/1
  purelin/1(a) -> Switch2/3, Fcn2/1
  Fcn2/1 -> Switch2/1
  Constant4/1 -> Switch2/2
  tansig/1(a) -> yhat1/1, Matrix Gain2/1
  Matrix Gain/1 -> netsum/2(In2)
  Matrix Gain1/1 -> netsum/1(In1)
  Constant/1 -> netsum/3(In3)
  netsum/1(Out1) -> tansig/1(n)
  Matrix Gain2/1 -> netsum1/1(In1)
  Constant1/1 -> netsum1/2(In2)
  netsum1/1(Out1) -> purelin/1(n)

== system neural/Control Systems/NARMA-L2 Controller/netsum ==
  In1 : Inport  Port=1  LatchInput=off
  In2 : Inport  Port=2  LatchInput=off
  netsum : Sum  Inputs=2  SaturateOnIntegerOverflow=on
  Out1 : Outport  Port=1
  wires:
  netsum/1 -> Out1/1
  In2/1 -> netsum/2
  In1/1 -> netsum/1

== system neural/Control Systems/NARMA-L2 Controller/netsum1 ==
  In1 : Inport  Port=1  LatchInput=off
  In2 : Inport  Port=2  LatchInput=off
  netsum1 : Sum  Inputs=2  SaturateOnIntegerOverflow=on
  Out1 : Outport  Port=1
  wires:
  netsum1/1 -> Out1/1
  In2/1 -> netsum1/2
  In1/1 -> netsum1/1

== system neural/Control Systems/NARMA-L2 Controller/netsum2 ==
  In1 : Inport  Port=1  LatchInput=off
  In2 : Inport  Port=2  LatchInput=off
  netsum : Sum  Inputs=2  SaturateOnIntegerOverflow=on
  Out1 : Outport  Port=1
  wires:
  netsum/1 -> Out1/1
  In2/1 -> netsum/2
  In1/1 -> netsum/1

== system neural/Control Systems/NARMA-L2 Controller/netsum3 ==
  In1 : Inport  Port=1  LatchInput=off
  In2 : Inport  Port=2  LatchInput=off
  netsum1 : Sum  Inputs=2  SaturateOnIntegerOverflow=on
  Out1 : Outport  Port=1
  wires:
  netsum1/1 -> Out1/1
  In2/1 -> netsum1/2
  In1/1 -> netsum1/1

== system neural/Control Systems/NARMA-L2 Controller/purelin ==
  n : Inport  Port=1  LatchInput=off
  a : Outport  Port=1
  wires:
  n/1 -> a/1

== system neural/Control Systems/NARMA-L2 Controller/purelin1 ==
  n : Inport  Port=1  LatchInput=off
  a : Outport  Port=1
  wires:
  n/1 -> a/1

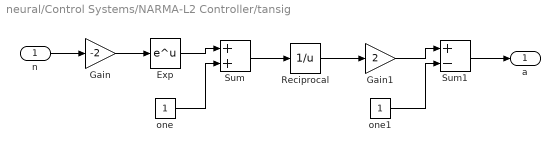
== system neural/Control Systems/NARMA-L2 Controller/tansig ==
  n : Inport  Port=1  LatchInput=off
  Exp : Math  Operator=exp  OutputSignalType=auto
  Gain : Gain  Gain=-2  Multiplication=Element-wise(K.*u)  SaturateOnIntegerOverflow=on
  Gain1 : Gain  Gain=2  Multiplication=Element-wise(K.*u)  SaturateOnIntegerOverflow=on
  Reciprocal : Math  Operator=reciprocal  OutputSignalType=auto
  Sum : Sum  Inputs=++  SaturateOnIntegerOverflow=on
  Sum1 : Sum  Inputs=+-  SaturateOnIntegerOverflow=on
  one : Constant  Value=1
  one1 : Constant  Value=1
  a : Outport  Port=1
  wires:
  Sum1/1 -> a/1
  one1/1 -> Sum1/2
  Gain1/1 -> Sum1/1
  Reciprocal/1 -> Gain1/1
  Sum/1 -> Reciprocal/1
  one/1 -> Sum/2
  Exp/1 -> Sum/1
  Gain/1 -> Exp/1
  n/1 -> Gain/1

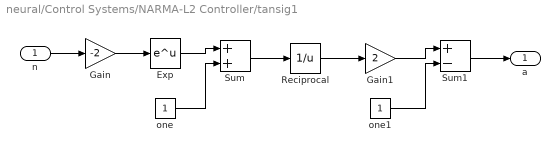
== system neural/Control Systems/NARMA-L2 Controller/tansig1 ==
  n : Inport  Port=1  LatchInput=off
  Exp : Math  Operator=exp  OutputSignalType=auto
  Gain : Gain  Gain=-2  Multiplication=Element-wise(K.*u)  SaturateOnIntegerOverflow=on
  Gain1 : Gain  Gain=2  Multiplication=Element-wise(K.*u)  SaturateOnIntegerOverflow=on
  Reciprocal : Math  Operator=reciprocal  OutputSignalType=auto
  Sum : Sum  Inputs=++  SaturateOnIntegerOverflow=on
  Sum1 : Sum  Inputs=+-  SaturateOnIntegerOverflow=on
  one : Constant  Value=1
  one1 : Constant  Value=1
  a : Outport  Port=1
  wires:
  Sum1/1 -> a/1
  one1/1 -> Sum1/2
  Gain1/1 -> Sum1/1
  Reciprocal/1 -> Gain1/1
  Sum/1 -> Reciprocal/1
  one/1 -> Sum/2
  Exp/1 -> Sum/1
  Gain/1 -> Exp/1
  n/1 -> Gain/1

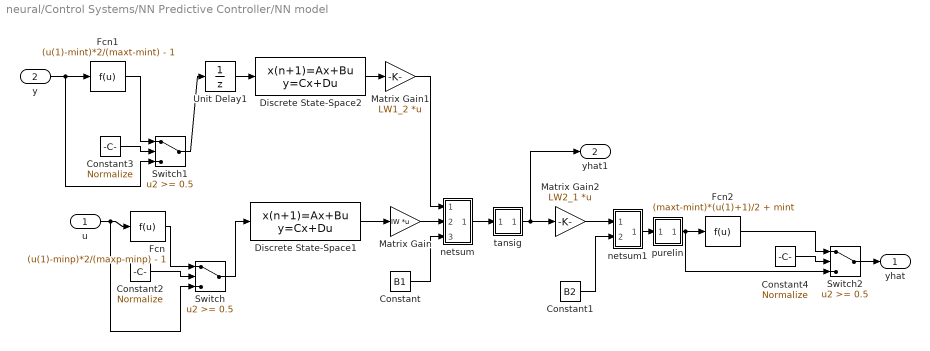
== system neural/Control Systems/NN Predictive Controller/NN model ==
  u : Inport  Port=1  LatchInput=off
  y : Inport  Port=2  LatchInput=off
  Constant : Constant  Value=B1
  Constant1 : Constant  Value=B2
  Constant2 : Constant  Value=Normalize
  Constant3 : Constant  Value=Normalize
  Constant4 : Constant  Value=Normalize
  Discrete State-Space1 : DiscreteStateSpace  A=[0 zeros(1,Ni-2);eye(Ni-2,Ni-1)]  B=[zeros(double(Ni==1));eye(Ni-1,1)]  C=[0 zeros(1,Ni-2);eye(Ni-1,Ni-1)]  D=eye(Ni,1)  X0=0  SampleTime=Ts  Realization=auto
      settings: RTWStateStorageClass=Auto
  Discrete State-Space2 : DiscreteStateSpace  A=[0 zeros(1,Nj-2);eye(Nj-2,Nj-1)]  B=[zeros(double(Nj==1));eye(Nj-1,1)]  C=[0 zeros(1,Nj-2);eye(Nj-1,Nj-1)]  D=eye(Nj,1)  X0=0  SampleTime=Ts  Realization=auto
      settings: RTWStateStorageClass=Auto
  Fcn : Fcn  Expr=(u(1)-minp)*2/(maxp-minp) - 1
  Fcn1 : Fcn  Expr=(u(1)-mint)*2/(maxt-mint) - 1
  Fcn2 : Fcn  Expr=(maxt-mint)*(u(1)+1)/2 + mint
  Matrix Gain : Gain  Gain=IW  Multiplication=Matrix(K*u)  SaturateOnIntegerOverflow=on
  Matrix Gain1 : Gain  Gain=LW1_2  Multiplication=Matrix(K*u)  SaturateOnIntegerOverflow=on
  Matrix Gain2 : Gain  Gain=LW2_1  Multiplication=Matrix(K*u)  SaturateOnIntegerOverflow=on
  Switch : Switch  Threshold=0.5  ZeroCross=off
  Switch1 : Switch  Threshold=0.5  ZeroCross=off
  Switch2 : Switch  Threshold=0.5  ZeroCross=off
  Unit Delay1 : UnitDelay  X0=0  SampleTime=Ts
      settings: RTWStateStorageClass=Auto
  netsum : Subsystem
      settings: RTWFcnNameOpts=Auto  RTWFileNameOpts=Auto
      mask Display: disp('+')
  netsum1 : Subsystem
      settings: RTWFcnNameOpts=Auto  RTWFileNameOpts=Auto
      mask Display: disp('+')
  purelin : Subsystem
      settings: RTWFcnNameOpts=Auto  RTWFileNameOpts=Auto
      mask Display: plot([-1 1],[0 0],[-1 1],[-1 1])
  tansig : Subsystem
      settings: RTWFcnNameOpts=Auto  RTWFileNameOpts=Auto
      mask Display: plot([-1 1],[0 0],[-1 -.9 -.8 -.7 -.6 -.5 -.4 -.3 -.2 -.1 0 .1 .2 .3 .4 .5 .6 .7 .8 .9 1],2./(1+exp(-8*[-1 -.9 -.8 -.7 -.6 -.5 -.4 -.3 -.2 -.1 0 .1 .2 .3 .4 .5 .6 .7 .8 .9 1]))-1)
  yhat : Outport  Port=1
  yhat1 : Outport  Port=2
  wires:
  netsum1/1(Out1) -> purelin/1(n)
  Constant1/1 -> netsum1/2(In2)
  Matrix Gain2/1 -> netsum1/1(In1)
  netsum/1(Out1) -> tansig/1(n)
  Constant/1 -> netsum/3(In3)
  Matrix Gain1/1 -> netsum/1(In1)
  Matrix Gain/1 -> netsum/2(In2)
  tansig/1(a) -> Matrix Gain2/1, yhat1/1
  Discrete State-Space1/1 -> Matrix Gain/1
  Fcn/1 -> Switch/1
  Switch/1 -> Discrete State-Space1/1
  u/1 -> Fcn/1, Switch/3
  Constant2/1 -> Switch/2
  Discrete State-Space2/1 -> Matrix Gain1/1
  Unit Delay1/1 -> Discrete State-Space2/1
  Constant3/1 -> Switch1/2
  Switch1/1 -> Unit Delay1/1
  Fcn1/1 -> Switch1/1
  y/1 -> Fcn1/1, Switch1/3
  Constant4/1 -> Switch2/2
  Switch2/1 -> yhat/1
  Fcn2/1 -> Switch2/1
  purelin/1(a) -> Fcn2/1, Switch2/3

== system neural/Weight Functions/dotprod/Dot Product ==
  in_1 : Inport  Port=1  LatchInput=off
  in_2 : Inport  Port=2  LatchInput=off
  Product : Product  Inputs=2  Multiplication=Element-wise(.*)  SaturateOnIntegerOverflow=on
  Sum : Sum  Inputs=+  SaturateOnIntegerOverflow=on
  out_1 : Outport  Port=1  InitialOutput=0
  wires:
  Sum/1 -> out_1/1
  Product/1 -> Sum/1
  in_1/1 -> Product/1
  in_2/1 -> Product/2

== system neural/Weight Functions/normprod/Dot Product ==
  in_1 : Inport  Port=1  LatchInput=off
  in_2 : Inport  Port=2  LatchInput=off
  Product : Product  Inputs=2  Multiplication=Element-wise(.*)  SaturateOnIntegerOverflow=on
  Sum : Sum  Inputs=+  SaturateOnIntegerOverflow=on
  out_1 : Outport  Port=1  InitialOutput=0
  wires:
  Sum/1 -> out_1/1
  Product/1 -> Sum/1
  in_1/1 -> Product/1
  in_2/1 -> Product/2

== system neural/Control Systems/Model Reference Controller/NN Controller/netsum ==
  In1 : Inport  Port=1  LatchInput=off
  In2 : Inport  Port=2  LatchInput=off
  In3 : Inport  Port=3  LatchInput=off
  In4 : Inport  Port=4  LatchInput=off
  netsum : Sum  Inputs=4  SaturateOnIntegerOverflow=on
  Out1 : Outport  Port=1
  wires:
  In4/1 -> netsum/4
  In3/1 -> netsum/3
  netsum/1 -> Out1/1
  In2/1 -> netsum/2
  In1/1 -> netsum/1

== system neural/Control Systems/Model Reference Controller/NN Controller/netsum1 ==
  In1 : Inport  Port=1  LatchInput=off
  In2 : Inport  Port=2  LatchInput=off
  netsum1 : Sum  Inputs=2  SaturateOnIntegerOverflow=on
  Out1 : Outport  Port=1
  wires:
  netsum1/1 -> Out1/1
  In2/1 -> netsum1/2
  In1/1 -> netsum1/1

== system neural/Control Systems/Model Reference Controller/NN Controller/purelin ==
  n : Inport  Port=1  LatchInput=off
  a : Outport  Port=1
  wires:
  n/1 -> a/1

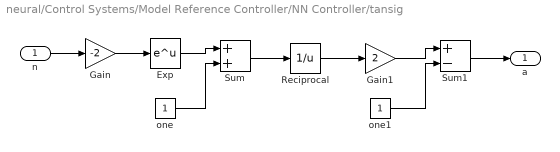
== system neural/Control Systems/Model Reference Controller/NN Controller/tansig ==
  n : Inport  Port=1  LatchInput=off
  Exp : Math  Operator=exp  OutputSignalType=auto
  Gain : Gain  Gain=-2  Multiplication=Element-wise(K.*u)  SaturateOnIntegerOverflow=on
  Gain1 : Gain  Gain=2  Multiplication=Element-wise(K.*u)  SaturateOnIntegerOverflow=on
  Reciprocal : Math  Operator=reciprocal  OutputSignalType=auto
  Sum : Sum  Inputs=++  SaturateOnIntegerOverflow=on
  Sum1 : Sum  Inputs=+-  SaturateOnIntegerOverflow=on
  one : Constant  Value=1
  one1 : Constant  Value=1
  a : Outport  Port=1
  wires:
  Sum1/1 -> a/1
  one1/1 -> Sum1/2
  Gain1/1 -> Sum1/1
  Reciprocal/1 -> Gain1/1
  Sum/1 -> Reciprocal/1
  one/1 -> Sum/2
  Exp/1 -> Sum/1
  Gain/1 -> Exp/1
  n/1 -> Gain/1

== system neural/Control Systems/Model Reference Controller/NN Plant/netsum ==
  In1 : Inport  Port=1  LatchInput=off
  In2 : Inport  Port=2  LatchInput=off
  In3 : Inport  Port=3  LatchInput=off
  netsum : Sum  Inputs=3  SaturateOnIntegerOverflow=on
  Out1 : Outport  Port=1
  wires:
  netsum/1 -> Out1/1
  In3/1 -> netsum/3
  In2/1 -> netsum/2
  In1/1 -> netsum/1

== system neural/Control Systems/Model Reference Controller/NN Plant/netsum1 ==
  In1 : Inport  Port=1  LatchInput=off
  In2 : Inport  Port=2  LatchInput=off
  netsum1 : Sum  Inputs=2  SaturateOnIntegerOverflow=on
  Out1 : Outport  Port=1
  wires:
  netsum1/1 -> Out1/1
  In2/1 -> netsum1/2
  In1/1 -> netsum1/1

== system neural/Control Systems/Model Reference Controller/NN Plant/purelin ==
  n : Inport  Port=1  LatchInput=off
  a : Outport  Port=1
  wires:
  n/1 -> a/1

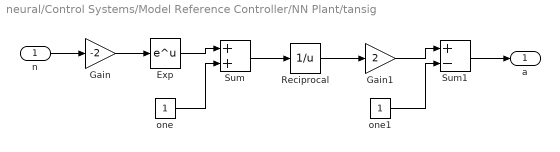
== system neural/Control Systems/Model Reference Controller/NN Plant/tansig ==
  n : Inport  Port=1  LatchInput=off
  Exp : Math  Operator=exp  OutputSignalType=auto
  Gain : Gain  Gain=-2  Multiplication=Element-wise(K.*u)  SaturateOnIntegerOverflow=on
  Gain1 : Gain  Gain=2  Multiplication=Element-wise(K.*u)  SaturateOnIntegerOverflow=on
  Reciprocal : Math  Operator=reciprocal  OutputSignalType=auto
  Sum : Sum  Inputs=++  SaturateOnIntegerOverflow=on
  Sum1 : Sum  Inputs=+-  SaturateOnIntegerOverflow=on
  one : Constant  Value=1
  one1 : Constant  Value=1
  a : Outport  Port=1
  wires:
  Sum1/1 -> a/1
  one1/1 -> Sum1/2
  Gain1/1 -> Sum1/1
  Reciprocal/1 -> Gain1/1
  Sum/1 -> Reciprocal/1
  one/1 -> Sum/2
  Exp/1 -> Sum/1
  Gain/1 -> Exp/1
  n/1 -> Gain/1

== system neural/Control Systems/NN Predictive Controller/NN model/netsum ==
  In1 : Inport  Port=1  LatchInput=off
  In2 : Inport  Port=2  LatchInput=off
  In3 : Inport  Port=3  LatchInput=off
  netsum : Sum  Inputs=3  SaturateOnIntegerOverflow=on
  Out1 : Outport  Port=1
  wires:
  In1/1 -> netsum/1
  In2/1 -> netsum/2
  In3/1 -> netsum/3
  netsum/1 -> Out1/1

== system neural/Control Systems/NN Predictive Controller/NN model/netsum1 ==
  In1 : Inport  Port=1  LatchInput=off
  In2 : Inport  Port=2  LatchInput=off
  netsum1 : Sum  Inputs=2  SaturateOnIntegerOverflow=on
  Out1 : Outport  Port=1
  wires:
  In1/1 -> netsum1/1
  In2/1 -> netsum1/2
  netsum1/1 -> Out1/1

== system neural/Control Systems/NN Predictive Controller/NN model/purelin ==
  n : Inport  Port=1  LatchInput=off
  a : Outport  Port=1
  wires:
  n/1 -> a/1

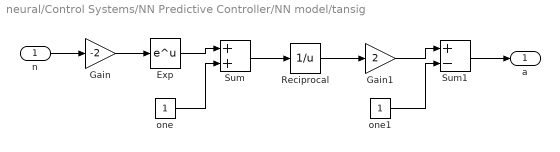
== system neural/Control Systems/NN Predictive Controller/NN model/tansig ==
  n : Inport  Port=1  LatchInput=off
  Exp : Math  Operator=exp  OutputSignalType=auto
  Gain : Gain  Gain=-2  Multiplication=Element-wise(K.*u)  SaturateOnIntegerOverflow=on
  Gain1 : Gain  Gain=2  Multiplication=Element-wise(K.*u)  SaturateOnIntegerOverflow=on
  Reciprocal : Math  Operator=reciprocal  OutputSignalType=auto
  Sum : Sum  Inputs=++  SaturateOnIntegerOverflow=on
  Sum1 : Sum  Inputs=+-  SaturateOnIntegerOverflow=on
  one : Constant  Value=1
  one1 : Constant  Value=1
  a : Outport  Port=1
  wires:
  n/1 -> Gain/1
  Gain/1 -> Exp/1
  Exp/1 -> Sum/1
  one/1 -> Sum/2
  Sum/1 -> Reciprocal/1
  Reciprocal/1 -> Gain1/1
  Gain1/1 -> Sum1/1
  one1/1 -> Sum1/2
  Sum1/1 -> a/1
